simulink model "mpc_project"  (R2023b)
settings: Solver=VariableStepAuto  StartTime=0.0  StopTime=15  RelTol=1e-3
values from neighbouring files (symbols this model uses):
  Ts = 0.02    [system_configuration.m]
  u_nom = 0    [system_configuration.m]
  y_nom = [0 0]    [system_configuration.m]
undefined symbols (not defined in the file or in its folder): a_max, T_regime, Td
libraries: cstblocks x2, mpclib x2
settings Model: Creator=aniello  LastModifiedBy=aniello

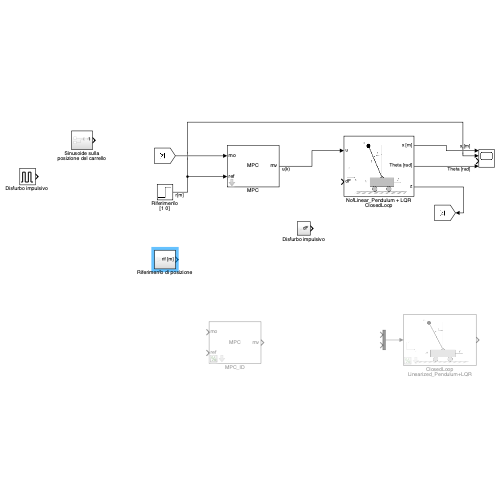
[thumbnail: Simulink's stored preview of the top-level diagram]
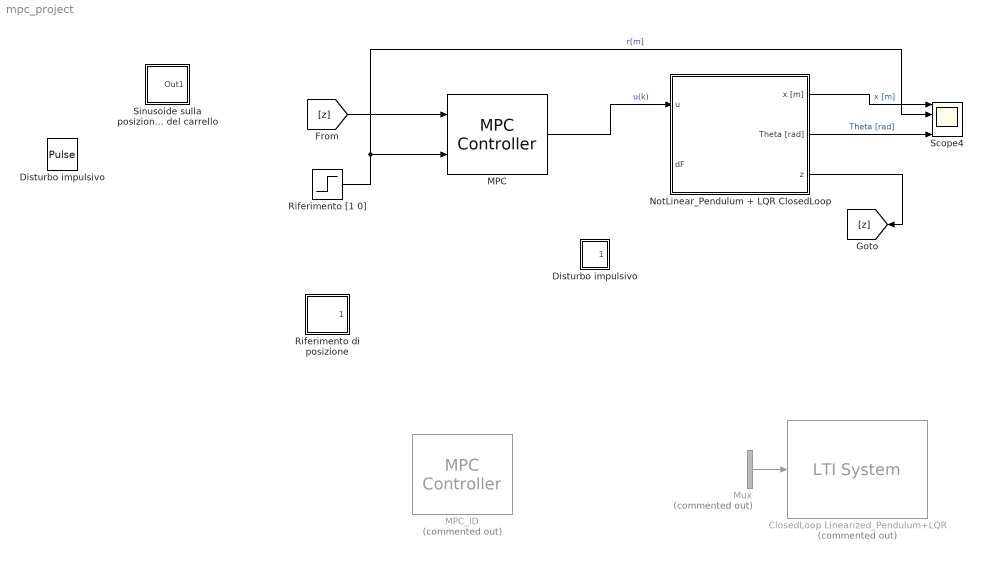
== system mpc_project ==
  ClosedLoop Linearized_Pendulum+LQR : cstblocks/LTI System  Commented=on  sys=F_k  IC=[]  PadeOrder=0  mask(LTI Block){}
      mask Display: image('pend_im.png');
  Disturbo impulsivo : Subsystem
  "Disturbo impulsivo " : DiscretePulseGenerator  PulseType=Time based  Amplitude=2  Period=8  PhaseDelay=8
  MPC : mpclib/MPC Controller  SCDEnableBlockLinearizationSpecification=on  mpcobj=mpc1  is_multiple=0  enable_value=0  return_u0=off  updateMPCinCallerWorkspace=on  md_inport=off  mv_inport=off  uref_inport=off  return_cost=off  return_mvseq=off  return_qpstatus=off  return_xseq=off  return_state=off  return_ovseq=off  state_inport=off  umin_inport=off  umax_inport=off  ymin_inport=off  ymax_inport=off  cc_inport=off  ywt_inport=off  uwt_inport=off  duwt_inport=off  rhoeps_inport=off  pm_inport=off  MaximumP=10  HorizonChoice=FixedHorizon  n_ts=0.02  n_p=40  n_mv=1  n_md=0  n_ud=1  n_mo=2  n_uo=0  BlockDataType=double  SampleTimeInherited=off  switch_inport=off
  MPC_ID : mpclib/MPC Controller  Commented=on  SCDEnableBlockLinearizationSpecification=on  mpcobj=mpc1_id  is_multiple=0  enable_value=0  return_u0=off  updateMPCinCallerWorkspace=on  md_inport=off  mv_inport=off  uref_inport=off  return_cost=off  return_mvseq=off  return_qpstatus=off  return_xseq=off  return_state=off  return_ovseq=off  state_inport=off  umin_inport=off  umax_inport=off  ymin_inport=off  ymax_inport=off  cc_inport=off  ywt_inport=off  uwt_inport=off  duwt_inport=off  rhoeps_inport=off  pm_inport=off  MaximumP=10  HorizonChoice=FixedHorizon  n_ts=0.02  n_p=40  n_mv=1  n_md=0  n_ud=1  n_mo=2  n_uo=0  BlockDataType=double  SampleTimeInherited=off  switch_inport=off
  Mux : Mux  Commented=on  Inputs=2
  NotLinear_Pendulum + LQR ClosedLoop : Subsystem
      mask Display: image('pend_im.png');
  Riferimento [1 0] : Step  Before=[0;0]  After=[1;0]  SampleTime=0
  Riferimento di posizione : Subsystem
  Scope4 : Scope  NumInputPorts=4
  Sinusoide sulla posizione del carrello : Subsystem
  wires:
  Mux/1 -> ClosedLoop Linearized_Pendulum+LQR/1
  NotLinear_Pendulum + LQR ClosedLoop/1(x [m]) -> Scope4/1  "x [m]"
  NotLinear_Pendulum + LQR ClosedLoop/2(Theta [rad]) -> Scope4/4  "Theta [rad]"
  NotLinear_Pendulum + LQR ClosedLoop/3(z) -> [z]
  Riferimento [1 0]/1 -> MPC/2, Scope4/2  "r[m]"
  [z] -> MPC/1
  MPC/1 -> NotLinear_Pendulum + LQR ClosedLoop/1(u)  "u(k)"

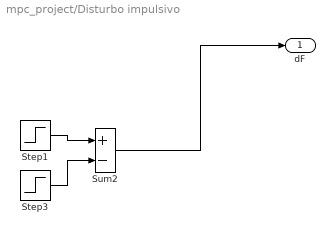
== system mpc_project/Disturbo impulsivo ==
  Step1 : Step  Time=8  SampleTime=0
  Step3 : Step  Time=8.04  SampleTime=0
  Sum2 : Sum  Inputs=+-
  dF : Outport
  wires:
  Sum2/1 -> dF/1
  Step3/1 -> Sum2/2
  Step1/1 -> Sum2/1

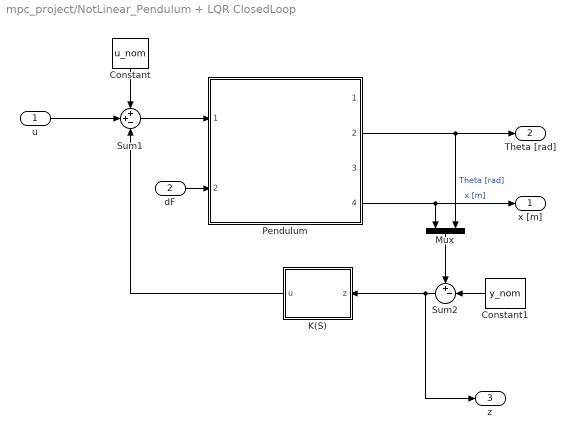
== system mpc_project/NotLinear_Pendulum + LQR ClosedLoop ==
  u : Inport
  dF : Inport  Port=2
  Constant : Constant  Value=u_nom
  Constant1 : Constant  Value=y_nom
  K(S) : Subsystem
  Mux : Mux  Inputs=2
  Pendulum : Subsystem  ReferencedSubsystem=pendulum
  Sum1 : Sum  Inputs=++-
  Sum2 : Sum  Inputs=+-|
  x [m] : Outport
  Theta [rad] : Outport  Port=2
  z : Outport  Port=3
  wires:
  K(S)/1(u) -> Sum1/3
  Mux/1 -> Sum2/1
  u/1 -> Sum1/2
  Sum2/1 -> z/1, K(S)/1(z)
  Constant/1 -> Sum1/1
  Constant1/1 -> Sum2/2
  Sum1/1 -> Pendulum/1
  Pendulum/2 -> Mux/2, Theta [rad]/1  "Theta [rad]"
  Pendulum/4 -> Mux/1, x [m]/1  "x [m]"
  dF/1 -> Pendulum/2

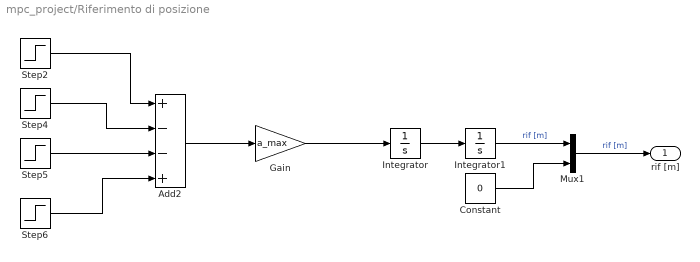
== system mpc_project/Riferimento di posizione ==
  Add2 : Sum  Inputs=+--+
  Constant : Constant  Value=0
  Gain : Gain  Gain=a_max
  Integrator : Integrator
  Integrator1 : Integrator
  Mux1 : Mux  Inputs=2
  Step2 : Step  SampleTime=0
  Step4 : Step  Time=Ts+1  SampleTime=0
  Step5 : Step  Time=Ts+T_regime+1  SampleTime=0
  Step6 : Step  Time=Ts+T_regime+Td+1  SampleTime=0
  rif [m] : Outport
  wires:
  Step6/1 -> Add2/4
  Step5/1 -> Add2/3
  Gain/1 -> Integrator/1
  Integrator/1 -> Integrator1/1
  Add2/1 -> Gain/1
  Step2/1 -> Add2/1
  Step4/1 -> Add2/2
  Mux1/1 -> rif [m]/1  "rif [m]"
  Constant/1 -> Mux1/2
  Integrator1/1 -> Mux1/1  "rif [m]"

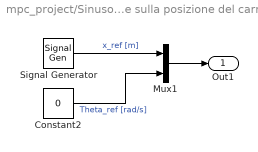
== system mpc_project/Sinusoide sulla posizione del carrello ==
  Constant2 : Constant  Value=0
  Mux1 : Mux  Inputs=2
  Signal Generator : SignalGenerator  Amplitude=2  Frequency=0.6  Units=rad/sec
  Out1 : Outport  Unit=m
  wires:
  Signal Generator/1 -> Mux1/1  "x_ref [m]"
  Constant2/1 -> Mux1/2  "Theta_ref [rad/s]"
  Mux1/1 -> Out1/1

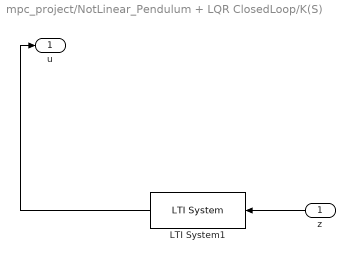
== system mpc_project/NotLinear_Pendulum + LQR ClosedLoop/K(S) ==
  z : Inport
  LTI System1 : cstblocks/LTI System  sys=K_s  IC=[]  PadeOrder=0
  u : Outport
  wires:
  LTI System1/1 -> u/1
  z/1 -> LTI System1/1
